simulink library "sharedTrackingLibrary"  (R2025a)
settings: Solver=VariableStepAuto  StartTime=0.0  StopTime=10.0  RelTol=1e-3
undefined symbols (not defined in the file): p
libraries: $bdroot x3
(part 2 of 2)

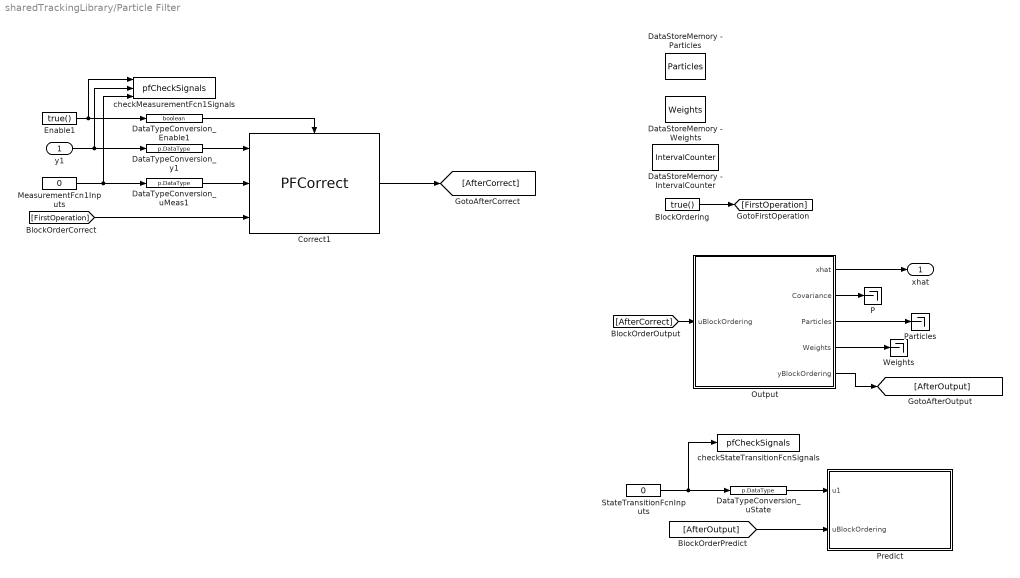
== system sharedTrackingLibrary/Particle Filter ==
  y1 : Inport
  BlockOrdering : Constant  Value=true()  OutDataTypeStr=boolean
  Correct1 : $bdroot/Extras/PFCorrect  ProcessedMaskData=p
  DataStoreMemory - IntervalCounter : DataStoreMemory  DataStoreName=IntervalCounter  VectorParams1D=off  ShowAdditionalParam=off  OutDataTypeStr=p.DataType
  DataStoreMemory - Particles : DataStoreMemory  DataStoreName=Particles  InitialValue=p.Particles  VectorParams1D=off  ShowAdditionalParam=off  OutDataTypeStr=p.DataType
  DataStoreMemory - Weights : DataStoreMemory  DataStoreName=Weights  InitialValue=p.Weights  VectorParams1D=off  ShowAdditionalParam=off  OutDataTypeStr=p.DataType
  DataTypeConversion_Enable1 : DataTypeConversion  OutDataTypeStr=boolean  SaturateOnIntegerOverflow=off  RndMeth=Floor
  DataTypeConversion_uMeas1 : DataTypeConversion  OutDataTypeStr=p.DataType  SaturateOnIntegerOverflow=off  RndMeth=Floor
  DataTypeConversion_uState : DataTypeConversion  OutDataTypeStr=p.DataType  SaturateOnIntegerOverflow=off  RndMeth=Floor
  DataTypeConversion_y1 : DataTypeConversion  OutDataTypeStr=p.DataType  SaturateOnIntegerOverflow=off  RndMeth=Floor
  Enable1 : Constant  Value=true()  SampleTime=p.SampleTimes.MeasurementFcn(1)
  MeasurementFcn1Inputs : Constant  Value=0  OutDataTypeStr=p.DataType  SampleTime=p.SampleTimes.MeasurementFcn(1)
  Output : Subsystem  TreatAsAtomicUnit=on  SystemSampleTime=p.SampleTimes.Output  mask{ProcessedMaskData=p}
      mask init:
      | if strcmp(get_param(bdroot,'SimulationStatus'),'stopped')
      |     pOutputs = [];
      | else
      |     pOutputs = ...
      |         matlabshared.tracking.internal.blocks.maskInitializationFcnPFOutputs(ProcessedMaskData);
      | end
  P : Terminator
  Particles : Terminator
  Predict : Subsystem  TreatAsAtomicUnit=on  SystemSampleTime=p.SampleTimes.StateTransitionFcn  mask(PFPredict){ProcessedMaskData=p}
      mask init:
      | if strcmp(get_param(bdroot,'SimulationStatus'),'stopped')
      |     pS = [];
      |     SampleTime = [];
      |     DataType = [];
      |     SLFcnsToRegister = {};
      | else
      |     [pS,SampleTime] = ...
      |         matlabshared.tracking.internal.blocks.maskInitializationFcnPFPredictor(ProcessedMaskData);
      |     [DataType,SLFcnsToRegister] = ...
      |         matlabshared.tracking.internal.blocks.maskInitializationFcnRegisterSLFcn(ProcessedMaskData, pS);
      | end
  StateTransitionFcnInputs : Constant  Value=0  OutDataTypeStr=p.DataType  SampleTime=p.SampleTimes.StateTransitionFcn
  Weights : Terminator
  checkMeasurementFcn1Signals : S-Function  FunctionName=pfCheckSignals  Parameters=signalCheck.BlockPath, signalCheck.MeasurementFcn{1}.PortNames, signalCheck.MeasurementFcn{1}.SampleTime, signalCheck.DataType, signalCheck.MeasurementFcn{1}.PortDimensions  SFunctionDeploymentMode=off  EnableBusSupport=off
  checkStateTransitionFcnSignals : S-Function  FunctionName=pfCheckSignals  Parameters=signalCheck.BlockPath, signalCheck.StateTransitionFcn.PortNames, signalCheck.StateTransitionFcn.SampleTime, signalCheck.DataType, signalCheck.StateTransitionFcn.PortDimensions  SFunctionDeploymentMode=off  EnableBusSupport=off
  xhat : Outport  VectorParamsAs1DForOutWhenUnconnected=off
  wires:
  [AfterCorrect] -> Output/1(uBlockOrdering)
  Correct1/1 -> [AfterCorrect]
  BlockOrdering/1 -> [FirstOperation]
  [FirstOperation] -> Correct1/3
  DataTypeConversion_y1/1 -> Correct1/1
  DataTypeConversion_uMeas1/1 -> Correct1/2
  Enable1/1 -> checkMeasurementFcn1Signals/1, DataTypeConversion_Enable1/1
  StateTransitionFcnInputs/1 -> checkStateTransitionFcnSignals/1, DataTypeConversion_uState/1
  MeasurementFcn1Inputs/1 -> checkMeasurementFcn1Signals/3, DataTypeConversion_uMeas1/1
  DataTypeConversion_uState/1 -> Predict/1(u1)
  DataTypeConversion_Enable1/1 -> Correct1/Enable
  Output/5(yBlockOrdering) -> [AfterOutput]
  Output/1(xhat) -> xhat/1
  Output/3(Particles) -> Particles/1
  Output/4(Weights) -> Weights/1
  Output/2(Covariance) -> P/1
  y1/1 -> DataTypeConversion_y1/1, checkMeasurementFcn1Signals/2
  [AfterOutput] -> Predict/2(uBlockOrdering)

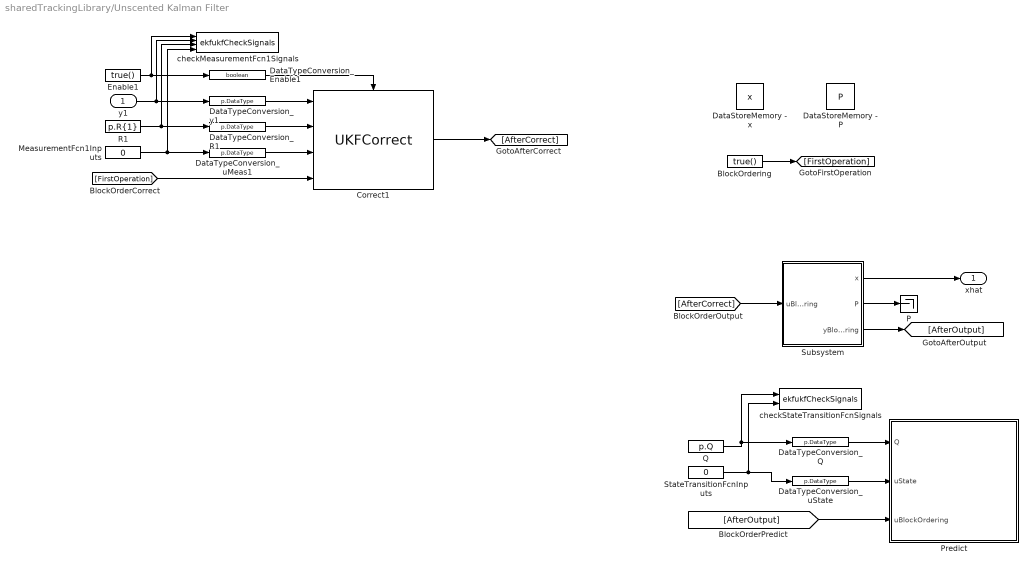
== system sharedTrackingLibrary/Unscented Kalman Filter ==
  y1 : Inport
  BlockOrdering : Constant  Value=true()  OutDataTypeStr=boolean
  Correct1 : $bdroot/Extras/UKFCorrect  ProcessedMaskData=p
  DataStoreMemory - P : DataStoreMemory  DataStoreName=P  InitialValue=p.InitialCovariance  ShowAdditionalParam=off  OutDataTypeStr=p.DataType
  DataStoreMemory - x : DataStoreMemory  DataStoreName=x  InitialValue=p.InitialState  ShowAdditionalParam=off  OutDataTypeStr=p.DataType
  DataTypeConversion_Enable1 : DataTypeConversion  OutDataTypeStr=boolean  SaturateOnIntegerOverflow=off  RndMeth=Floor
  DataTypeConversion_Q : DataTypeConversion  OutDataTypeStr=p.DataType  SaturateOnIntegerOverflow=off  RndMeth=Floor
  DataTypeConversion_R1 : DataTypeConversion  OutDataTypeStr=p.DataType  SaturateOnIntegerOverflow=off  RndMeth=Floor
  DataTypeConversion_uMeas1 : DataTypeConversion  OutDataTypeStr=p.DataType  SaturateOnIntegerOverflow=off  RndMeth=Floor
  DataTypeConversion_uState : DataTypeConversion  OutDataTypeStr=p.DataType  SaturateOnIntegerOverflow=off  RndMeth=Floor
  DataTypeConversion_y1 : DataTypeConversion  OutDataTypeStr=p.DataType  SaturateOnIntegerOverflow=off  RndMeth=Floor
  Enable1 : Constant  Value=true()  SampleTime=p.SampleTimes.MeasurementFcn(1)
  MeasurementFcn1Inputs : Constant  Value=0  OutDataTypeStr=p.DataType  SampleTime=p.SampleTimes.MeasurementFcn(1)
  P : Terminator
  Predict : Subsystem  TreatAsAtomicUnit=on  SystemSampleTime=p.SampleTimes.StateTransitionFcn  mask(UKFPredict){ProcessedMaskData=p}
      mask init:
      | if strcmp(get_param(bdroot,'SimulationStatus'),'stopped')
      |     pS = [];
      |     SampleTime = [];
      |     DataType = [];
      |     SLFcnsToRegister = {};
      | else
      |     [pS,SampleTime] = ...
      |         matlabshared.tracking.internal.blocks.maskInitializationFcnUKFPredictor(ProcessedMaskData);
      |     [DataType,SLFcnsToRegister] = ...
      |         matlabshared.tracking.internal.blocks.maskInitializationFcnRegisterSLFcn(ProcessedMaskData, pS);
      | end
  Q : Constant  Value=p.Q  SampleTime=p.SampleTimes.StateTransitionFcn
  R1 : Constant  Value=p.R{1}  SampleTime=p.SampleTimes.MeasurementFcn(1)
  StateTransitionFcnInputs : Constant  Value=0  OutDataTypeStr=p.DataType  SampleTime=p.SampleTimes.StateTransitionFcn
  Subsystem : Subsystem  TreatAsAtomicUnit=on  SystemSampleTime=p.SampleTimes.Output
  checkMeasurementFcn1Signals : S-Function  FunctionName=ekfukfCheckSignals  Parameters=signalCheck.BlockPath, signalCheck.MeasurementFcn{1}.PortNames, signalCheck.MeasurementFcn{1}.SampleTime, signalCheck.DataType, signalCheck.MeasurementFcn{1}.PortDimensions, 1, signalCheck.MeasurementFcn{1}.HasAdditiveNoise  SFunctionDeploymentMode=off  EnableBusSupport=off
  checkStateTransitionFcnSignals : S-Function  FunctionName=ekfukfCheckSignals  Parameters=signalCheck.BlockPath, signalCheck.StateTransitionFcn.PortNames, signalCheck.StateTransitionFcn.SampleTime, signalCheck.DataType, signalCheck.StateTransitionFcn.PortDimensions, 0, signalCheck.StateTransitionFcn.HasAdditiveNoise  SFunctionDeploymentMode=off  EnableBusSupport=off
  xhat : Outport  VectorParamsAs1DForOutWhenUnconnected=off
  wires:
  BlockOrdering/1 -> [FirstOperation]
  [FirstOperation] -> Correct1/4
  DataTypeConversion_y1/1 -> Correct1/1
  y1/1 -> checkMeasurementFcn1Signals/2, DataTypeConversion_y1/1
  R1/1 -> checkMeasurementFcn1Signals/3, DataTypeConversion_R1/1
  DataTypeConversion_uMeas1/1 -> Correct1/3
  Enable1/1 -> checkMeasurementFcn1Signals/1, DataTypeConversion_Enable1/1
  StateTransitionFcnInputs/1 -> checkStateTransitionFcnSignals/2, DataTypeConversion_uState/1
  MeasurementFcn1Inputs/1 -> checkMeasurementFcn1Signals/4, DataTypeConversion_uMeas1/1
  DataTypeConversion_R1/1 -> Correct1/2
  DataTypeConversion_uState/1 -> Predict/2(uState)
  Q/1 -> checkStateTransitionFcnSignals/1, DataTypeConversion_Q/1
  DataTypeConversion_Enable1/1 -> Correct1/Enable
  DataTypeConversion_Q/1 -> Predict/1(Q)
  [AfterCorrect] -> Subsystem/1(uBlockOrdering)
  Subsystem/1(x) -> xhat/1
  Subsystem/2(P) -> P/1
  Subsystem/3(yBlockOrdering) -> [AfterOutput]
  Correct1/1 -> [AfterCorrect]
  [AfterOutput] -> Predict/3(uBlockOrdering)

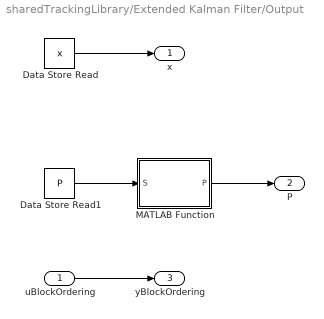
== system sharedTrackingLibrary/Extended Kalman Filter/Output ==
  uBlockOrdering : Inport
  Data Store Read : DataStoreRead  DataStoreName=x  IndexOptions=Index vector (dialog)  Indices=1  OutputSizes=1
  Data Store Read1 : DataStoreRead  DataStoreName=P  IndexOptions=Index vector (dialog)  Indices=1  OutputSizes=1
  MATLAB Function : MATLAB Function  TreatAsAtomicUnit=on
  x : Outport  VectorParamsAs1DForOutWhenUnconnected=off
  P : Outport  Port=2  VectorParamsAs1DForOutWhenUnconnected=off
  yBlockOrdering : Outport  Port=3  VectorParamsAs1DForOutWhenUnconnected=off
  wires:
  Data Store Read/1 -> x/1
  Data Store Read1/1 -> MATLAB Function/1(S)
  uBlockOrdering/1 -> yBlockOrdering/1
  MATLAB Function/1(P) -> P/1

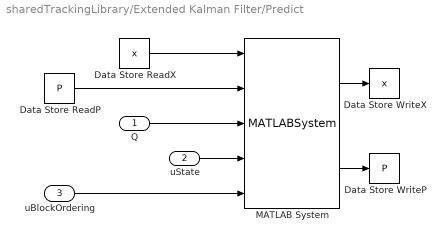
== system sharedTrackingLibrary/Extended Kalman Filter/Predict ==
  Q : Inport  SampleTime=SampleTime
  uState : Inport  Port=2  SampleTime=SampleTime
  uBlockOrdering : Inport  Port=3  SampleTime=SampleTime
  Data Store WriteP : DataStoreWrite  DataStoreName=P  IndexOptions=Index vector (dialog)  Indices=1  OutputSizes=1
  Data Store WriteX : DataStoreWrite  DataStoreName=x  IndexOptions=Index vector (dialog)  Indices=1  OutputSizes=1
  Data Store ReadP : DataStoreRead  DataStoreName=P  IndexOptions=Index vector (dialog)  Indices=1  OutputSizes=1
  Data Store ReadX : DataStoreRead  DataStoreName=x  IndexOptions=Index vector (dialog)  Indices=1  OutputSizes=1
  MATLAB System : MATLABSystem  System=matlabshared.tracking.internal.blocks.ekfPredictFcn  DlgParamStruct=pS  SLFcn=SLFcnsToRegister  DataType=DataType  SimulateUsing=Code generation
      mask Type: matlabshared.tracking.internal.blocks.ekfPredictFcn
  wires:
  Data Store ReadP/1 -> MATLAB System/2
  MATLAB System/2 -> Data Store WriteP/1
  Q/1 -> MATLAB System/3
  MATLAB System/1 -> Data Store WriteX/1
  Data Store ReadX/1 -> MATLAB System/1
  uState/1 -> MATLAB System/4
  uBlockOrdering/1 -> MATLAB System/5

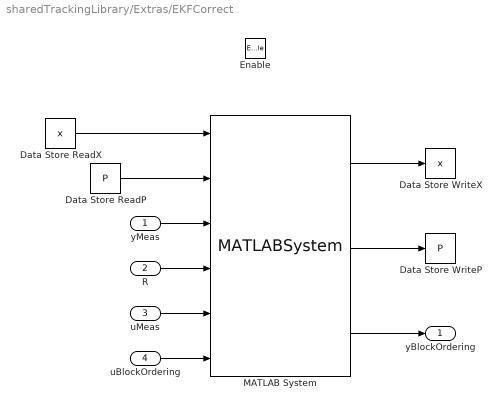
== system sharedTrackingLibrary/Extras/EKFCorrect ==
  yMeas : Inport  SampleTime=SampleTime
  R : Inport  Port=2  SampleTime=SampleTime
  uMeas : Inport  Port=3  SampleTime=SampleTime
  uBlockOrdering : Inport  Port=4  SampleTime=SampleTime
  Enable : EnablePort
  Data Store ReadP : DataStoreRead  DataStoreName=P  IndexOptions=Index vector (dialog)  Indices=1  OutputSizes=1
  Data Store ReadX : DataStoreRead  DataStoreName=x  IndexOptions=Index vector (dialog)  Indices=1  OutputSizes=1
  Data Store WriteP : DataStoreWrite  DataStoreName=P  IndexOptions=Index vector (dialog)  Indices=1  OutputSizes=1
  Data Store WriteX : DataStoreWrite  DataStoreName=x  IndexOptions=Index vector (dialog)  Indices=1  OutputSizes=1
  MATLAB System : MATLABSystem  System=matlabshared.tracking.internal.blocks.ekfCorrectFcn  DlgParamStruct=pM  SLFcn=SLFcnsToRegister  DataType=DataType  SampleTime=SampleTime  SimulateUsing=Code generation
      mask Type: matlabshared.tracking.internal.blocks.ekfCorrectFcn
  yBlockOrdering : Outport  VectorParamsAs1DForOutWhenUnconnected=off
  wires:
  Data Store ReadX/1 -> MATLAB System/1
  Data Store ReadP/1 -> MATLAB System/2
  MATLAB System/2 -> Data Store WriteP/1
  yMeas/1 -> MATLAB System/3
  R/1 -> MATLAB System/4
  MATLAB System/1 -> Data Store WriteX/1
  MATLAB System/3 -> yBlockOrdering/1
  uBlockOrdering/1 -> MATLAB System/6
  uMeas/1 -> MATLAB System/5

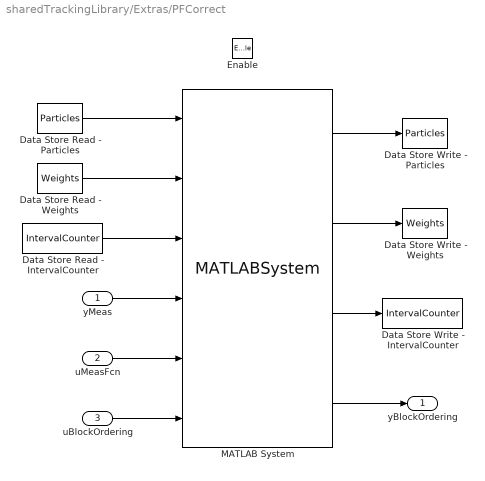
== system sharedTrackingLibrary/Extras/PFCorrect ==
  yMeas : Inport  SampleTime=SampleTime
  uMeasFcn : Inport  Port=2  SampleTime=SampleTime
  uBlockOrdering : Inport  Port=3  SampleTime=SampleTime
  Enable : EnablePort
  Data Store Read - IntervalCounter : DataStoreRead  DataStoreName=IntervalCounter  IndexOptions=Index vector (dialog)  Indices=1  OutputSizes=1
  Data Store Read - Particles : DataStoreRead  DataStoreName=Particles  IndexOptions=Index vector (dialog)  Indices=1  OutputSizes=1
  Data Store Read - Weights : DataStoreRead  DataStoreName=Weights  IndexOptions=Index vector (dialog)  Indices=1  OutputSizes=1
  Data Store Write - IntervalCounter : DataStoreWrite  DataStoreName=IntervalCounter  IndexOptions=Index vector (dialog)  Indices=1  OutputSizes=1
  Data Store Write - Particles : DataStoreWrite  DataStoreName=Particles  IndexOptions=Index vector (dialog)  Indices=1  OutputSizes=1
  Data Store Write - Weights : DataStoreWrite  DataStoreName=Weights  IndexOptions=Index vector (dialog)  Indices=1  OutputSizes=1
  MATLAB System : MATLABSystem  System=matlabshared.tracking.internal.blocks.pfCorrectFcn  DlgParamStruct=pM  SLFcn=pRegisterSLFcn.SLFcnsToRegister  DataType=pRegisterSLFcn.DataType  SampleTime=SampleTime  SimulateUsing=Code generation
      mask Type: matlabshared.tracking.internal.blocks.pfCorrectFcn
  yBlockOrdering : Outport  VectorParamsAs1DForOutWhenUnconnected=off
  wires:
  Data Store Read - Particles/1 -> MATLAB System/1
  yMeas/1 -> MATLAB System/4
  MATLAB System/1 -> Data Store Write - Particles/1
  uBlockOrdering/1 -> MATLAB System/6
  MATLAB System/4 -> yBlockOrdering/1
  Data Store Read - Weights/1 -> MATLAB System/2
  MATLAB System/2 -> Data Store Write - Weights/1
  MATLAB System/3 -> Data Store Write - IntervalCounter/1
  Data Store Read - IntervalCounter/1 -> MATLAB System/3
  uMeasFcn/1 -> MATLAB System/5

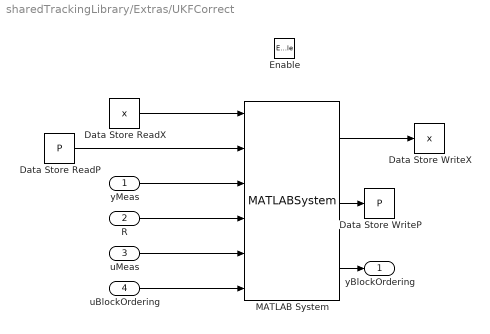
== system sharedTrackingLibrary/Extras/UKFCorrect ==
  yMeas : Inport  SampleTime=SampleTime
  R : Inport  Port=2  SampleTime=SampleTime
  uMeas : Inport  Port=3  SampleTime=SampleTime
  uBlockOrdering : Inport  Port=4  SampleTime=SampleTime
  Enable : EnablePort
  Data Store WriteP : DataStoreWrite  DataStoreName=P  IndexOptions=Index vector (dialog)  Indices=1  OutputSizes=1
  Data Store WriteX : DataStoreWrite  DataStoreName=x  IndexOptions=Index vector (dialog)  Indices=1  OutputSizes=1
  Data Store ReadP : DataStoreRead  DataStoreName=P  IndexOptions=Index vector (dialog)  Indices=1  OutputSizes=1
  Data Store ReadX : DataStoreRead  DataStoreName=x  IndexOptions=Index vector (dialog)  Indices=1  OutputSizes=1
  MATLAB System : MATLABSystem  System=matlabshared.tracking.internal.blocks.ukfCorrectFcn  DlgParamStruct=pM  SLFcn=SLFcnsToRegister  DataType=DataType  SampleTime=SampleTime  SimulateUsing=Code generation
      mask Type: matlabshared.tracking.internal.blocks.ukfCorrectFcn
  yBlockOrdering : Outport  VectorParamsAs1DForOutWhenUnconnected=off
  wires:
  Data Store ReadX/1 -> MATLAB System/1
  Data Store ReadP/1 -> MATLAB System/2
  MATLAB System/2 -> Data Store WriteP/1
  yMeas/1 -> MATLAB System/3
  R/1 -> MATLAB System/4
  MATLAB System/1 -> Data Store WriteX/1
  uBlockOrdering/1 -> MATLAB System/6
  MATLAB System/3 -> yBlockOrdering/1
  uMeas/1 -> MATLAB System/5

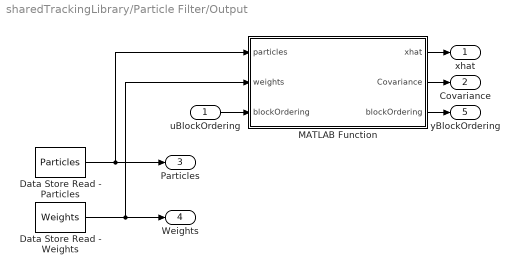
== system sharedTrackingLibrary/Particle Filter/Output ==
  uBlockOrdering : Inport
  Data Store Read - Particles : DataStoreRead  DataStoreName=Particles  IndexOptions=Index vector (dialog)  Indices=1  OutputSizes=1
  Data Store Read - Weights : DataStoreRead  DataStoreName=Weights  IndexOptions=Index vector (dialog)  Indices=1  OutputSizes=1
  MATLAB Function : MATLAB Function  TreatAsAtomicUnit=on
  xhat : Outport  VectorParamsAs1DForOutWhenUnconnected=off
  Covariance : Outport  Port=2  VectorParamsAs1DForOutWhenUnconnected=off
  Particles : Outport  Port=3  VectorParamsAs1DForOutWhenUnconnected=off
  Weights : Outport  Port=4  VectorParamsAs1DForOutWhenUnconnected=off
  yBlockOrdering : Outport  Port=5  VectorParamsAs1DForOutWhenUnconnected=off
  wires:
  Data Store Read - Weights/1 -> Weights/1, MATLAB Function/2(weights)
  Data Store Read - Particles/1 -> MATLAB Function/1(particles), Particles/1
  MATLAB Function/2(Covariance) -> Covariance/1
  MATLAB Function/1(xhat) -> xhat/1
  uBlockOrdering/1 -> MATLAB Function/3("blockOrdering ")
  MATLAB Function/3(blockOrdering) -> yBlockOrdering/1

== system sharedTrackingLibrary/Particle Filter/Predict ==
  u1 : Inport  SampleTime=SampleTime
  uBlockOrdering : Inport  Port=2
  Data Store Read - Particles : DataStoreRead  DataStoreName=Particles  IndexOptions=Index vector (dialog)  Indices=1  OutputSizes=1
  Data Store Write - Particles : DataStoreWrite  DataStoreName=Particles  IndexOptions=Index vector (dialog)  Indices=1  OutputSizes=1
  MATLAB System : MATLABSystem  System=matlabshared.tracking.internal.blocks.pfPredictFcn  DlgParamStruct=pS  SLFcn=SLFcnsToRegister  DataType=DataType  SimulateUsing=Code generation
      mask Type: matlabshared.tracking.internal.blocks.pfPredictFcn
  wires:
  MATLAB System/1 -> Data Store Write - Particles/1
  Data Store Read - Particles/1 -> MATLAB System/1
  u1/1 -> MATLAB System/2
  uBlockOrdering/1 -> MATLAB System/3

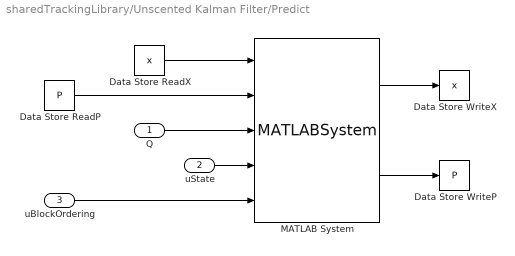
== system sharedTrackingLibrary/Unscented Kalman Filter/Predict ==
  Q : Inport  SampleTime=SampleTime
  uState : Inport  Port=2  SampleTime=SampleTime
  uBlockOrdering : Inport  Port=3
  Data Store WriteP : DataStoreWrite  DataStoreName=P  IndexOptions=Index vector (dialog)  Indices=1  OutputSizes=1
  Data Store WriteX : DataStoreWrite  DataStoreName=x  IndexOptions=Index vector (dialog)  Indices=1  OutputSizes=1
  Data Store ReadP : DataStoreRead  DataStoreName=P  IndexOptions=Index vector (dialog)  Indices=1  OutputSizes=1
  Data Store ReadX : DataStoreRead  DataStoreName=x  IndexOptions=Index vector (dialog)  Indices=1  OutputSizes=1
  MATLAB System : MATLABSystem  System=matlabshared.tracking.internal.blocks.ukfPredictFcn  DlgParamStruct=pS  SLFcn=SLFcnsToRegister  DataType=DataType  SimulateUsing=Code generation
      mask Type: matlabshared.tracking.internal.blocks.ukfPredictFcn
  wires:
  Data Store ReadP/1 -> MATLAB System/2
  MATLAB System/2 -> Data Store WriteP/1
  Q/1 -> MATLAB System/3
  MATLAB System/1 -> Data Store WriteX/1
  Data Store ReadX/1 -> MATLAB System/1
  uState/1 -> MATLAB System/4
  uBlockOrdering/1 -> MATLAB System/5

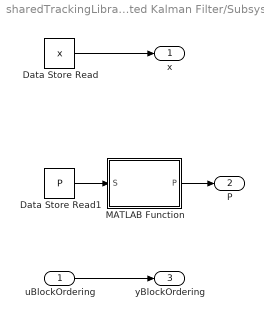
== system sharedTrackingLibrary/Unscented Kalman Filter/Subsystem ==
  uBlockOrdering : Inport
  Data Store Read : DataStoreRead  DataStoreName=x  IndexOptions=Index vector (dialog)  Indices=1  OutputSizes=1
  Data Store Read1 : DataStoreRead  DataStoreName=P  IndexOptions=Index vector (dialog)  Indices=1  OutputSizes=1
  MATLAB Function : MATLAB Function  TreatAsAtomicUnit=on
  x : Outport  VectorParamsAs1DForOutWhenUnconnected=off
  P : Outport  Port=2  VectorParamsAs1DForOutWhenUnconnected=off
  yBlockOrdering : Outport  Port=3  VectorParamsAs1DForOutWhenUnconnected=off
  wires:
  Data Store Read/1 -> x/1
  Data Store Read1/1 -> MATLAB Function/1(S)
  uBlockOrdering/1 -> yBlockOrdering/1
  MATLAB Function/1(P) -> P/1

== matlab function sharedTrackingLibrary/Extended Kalman Filter/Output/MATLAB Function ==
  data: S input; P output
function P = fcn(S)
    
    % Get back Covariance from Square-root Covariance
    P = S*S';
    
end

== matlab function sharedTrackingLibrary/Unscented Kalman Filter/Subsystem/MATLAB Function ==
  data: S input; P output
function P = fcn(S)
    
    % Get back Covariance from Square-root Covariance
    P = S*S';
    
end

== matlab function sharedTrackingLibrary/Particle Filter/Output/MATLAB Function ==
  data: particles input; weights input; blockOrdering input; pOutputs parameter; xhat output; Covariance output; blockOrdering output
function [xhat,Covariance,blockOrdering] = ...
    calculateStateAndCovariance(particles,weights,blockOrdering,pOutputs)

%% Quick return if no work is needed
if strcmp(pOutputs.StateEstimationMethod,'none')
    xhat = cast(0,'like',particles);
    Covariance = cast(0,'like',particles);
    return;
end

%% Preparation
% Get the state estimator object
switch pOutputs.StateEstimationMethod
    case 'mean'
        stateEstimator = matlabshared.tracking.internal.MeanStateEstimator;
        OutputState = true();
        OutputCov = pOutputs.OutputStateCovariance; % Follow user's preference
    case 'maxweight'
        stateEstimator = matlabshared.tracking.internal.MaxWeightStateEstimator;
        OutputState = true();
        OutputCov = false(); % No covariance to output, even if user requested
    case 'none'
        % This code path should never be reached due to quick return code
        % in the beginnin
        stateEstimator = cast(0,'like',particles);
        OutputState = false();
        OutputCov = false();
    otherwise
        assert(false);
end
% Get the particle manager
particleManager = matlabshared.tracking.internal.ParticleFilter.initializeParticleManager(pOutputs.IsStateOrientationColumn);

%% Results
% At least 1 output was requested (Covariance or xhat)   
if OutputCov
    % xhat is calculated in the process of calculating Covariance. No need
    % to check if xhat was requested or not. Block will not show an outport
    % if xhat was not requested.
    [xhat,Covariance] = stateEstimator.estimate(particleManager, particles,...
        weights, pOutputs.IsStateVariableCircular);
elseif OutputState
    % xhat was requested, but not the covariance. 
    xhat = stateEstimator.estimate(particleManager, particles, weights,...
        pOutputs.IsStateVariableCircular);
    Covariance = cast(0,'like',particles);
else
    xhat = cast(0,'like',particles);
    Covariance = cast(0,'like',particles);
end

end
